simulink model "section_E"  (R2023b)
settings: Solver=VariableStepAuto  StartTime=0.0  StopTime=100000000  RelTol=1e-3
values from neighbouring files (symbols this model uses):
  k = 4    [data.mat]    (also in section_E_script.m = ks(i))
  n = 7    [data.mat]    (also in section_E_script.m = ns(i))
libraries: commdigbbndpm3 x2, commblkcod2 x2, commchan3 x1, commsink2 x1, commrandsrc3 x1

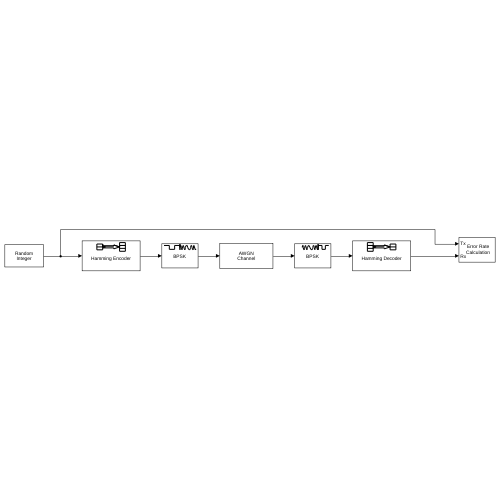
[thumbnail: Simulink's stored preview of the top-level diagram]
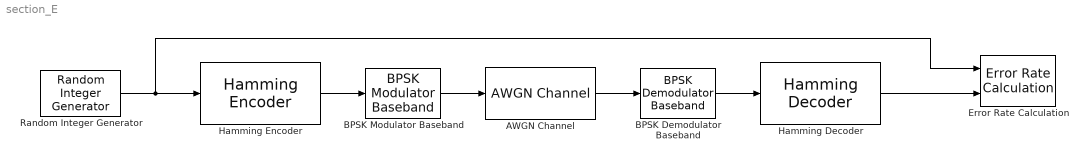
== system section_E ==
  AWGN Channel : commchan3/AWGN Channel  LegacyMode=off  NoiseMethod="Signal to noise ratio  (Eb/No)"  noiseMode="Signal to noise ratio  (SNR)"  EbNo=Eb_N0_in_dB  EsNo=10  SNR=10  BitsPerSymbol=1  SignalPower=1  SamplesPerSymbol=1  SymbolPeriod=1  VarianceSource=Parameter  Variance=1  RandomStream=Global stream  Seed=67  SimulateUsing=Code generation
  BPSK Demodulator Baseband : commdigbbndpm3/BPSK Demodulator Baseband  DecType=Hard decision  VarSource=Dialog  Variance=1  Ph=0  outDtype=Inherit via internal rule  derotateFactorWordLen=16  derotateFactorDataTypeStr=Inherit: Same word length as input  derotateFactorLastDataTypeStr=Inherit: Same word length as input
  BPSK Modulator Baseband : commdigbbndpm3/BPSK Modulator Baseband  Ph=0  outDtype=double  outWordLen=16  outUDDataType=sfix(16)  outFracLenMode=Best precision  outFracLen=15  outDataTypeStr=double  outLastDataTypeStr=double
  Error Rate Calculation : commsink2/Error Rate Calculation  N=0  st_delay=0  cp_mode=Entire frame  subframe=[]  PMode=Workspace  WsName=ErrorVec  RsMode2=off  stop=on  numErr=1000  maxBits=1e9
  Hamming Decoder : commblkcod2/Hamming Decoder  n=n  k=k
  Hamming Encoder : commblkcod2/Hamming Encoder  n=n  k=k
  Random Integer Generator : commrandsrc3/Random Integer Generator  SetSize=2  SeedSource=Auto  Seed=0  SampleTime=n/k  SamplesPerFrame=k  OutputDataType=double  SimulateUsing=Interpreted execution
  wires:
  Random Integer Generator/1 -> Error Rate Calculation/1, Hamming Encoder/1
  Hamming Encoder/1 -> BPSK Modulator Baseband/1
  BPSK Modulator Baseband/1 -> AWGN Channel/1
  AWGN Channel/1 -> BPSK Demodulator Baseband/1
  BPSK Demodulator Baseband/1 -> Hamming Decoder/1
  Hamming Decoder/1 -> Error Rate Calculation/2
